simulink model "numerical_model"  (R2021a)
settings: Solver=VariableStepAuto  StartTime=0.0  StopTime=100  RelTol=1e-6
values from neighbouring files (symbols this model uses):
  d_f = 0.1*[1 1 1].'    [working_numerlical_sim_sys_param.m]
  d_tau = 0.1*[1 1 1].'    [working_numerlical_sim_sys_param.m]
  g = 9.81    [working_numerlical_sim_sys_param.m]
  Gamma = 0.1*eye(6)    [working_numerlical_sim_sys_param.m]
  J = [0.0169572, 0 0; 0 0.0169572 0; 0 0 0.0338078]    [working_numerlical_sim_sys_param.m]
  Jv0 = 0.8*[J(1,1) J(2,2) J(3,3) J(1,2) J(2,3) J(1,3)].'    [working_numerlical_sim_sys_param.m]
  k1 = 0.4    [working_numerlical_sim_sys_param.m]
  k2 = 0.5    [working_numerlical_sim_sys_param.m]
  k3 = 0.5    [working_numerlical_sim_sys_param.m]
  k4 = 2    [working_numerlical_sim_sys_param.m]
  k5 = 1    [working_numerlical_sim_sys_param.m]
  k_dtau = 1    [working_numerlical_sim_sys_param.m]
  k_psi1 = 1    [working_numerlical_sim_sys_param.m]
  k_psi2 = 1    [working_numerlical_sim_sys_param.m]
  lambda = 86    [working_numerlical_sim_sys_param.m]
  m = quadrotor_mass+link0_mass+link1_mass    (= 1.8)    [working_numerlical_sim_sys_param.m]
  m0 = 0.9*m    (= 1.62)    [working_numerlical_sim_sys_param.m]
  omega_0 = 0*[0.1 -0.1 0.1].'    [working_numerlical_sim_sys_param.m]
  p_0 = [-0.1 0.1 -0.9].'    [working_numerlical_sim_sys_param.m]
  R_0 = eye(3)    [working_numerlical_sim_sys_param.m]
  v_0 = [0 0 0].'    [working_numerlical_sim_sys_param.m]
settings Model: Creator=Awais  LastModifiedBy=awais
settings SolverCC: AlgebraicLoopSolver=TrustRegion
settings DebuggingCC: SFMachineParentedDataDiag=warning
settings ExplorerConfigSet: InternalSimMechanicsExplorerSettings="<ExplorerConfiguration><canonicalview>aerospace</canonicalview><AnimationSetting><BasePlaybackSpeed>1.0</BasePlaybackSpeed><PlaybackSpeedFactor>1.0</PlaybackSpeedFactor></AnimationSetting><TilePanel><TileInfo><Tiles Columns=\"1\" Count=\"1\" Rows=\"1\"><Column Weight=\"1\"/><Row Weight=\"1\"/><Tile Height=\"1\" Width=\"1\" X=\"0\" Y=\"0\"/></Tiles></TileInfo><SceneInfo><SceneViewer><BGColor><R>1</R><G>1</G><B>1</B></BGColor><Camera><DoPerspective>off</DoPerspective><Position><X>9.64020367718573112</X><Y>-9.14802033169267048</Y><Z>-6.8961967369270063</Z></Position><Center><X>1.75390707402820034</X><Y>-2.22859187648804102</Y><Z>3.98852762898917668</Z></Center><Up><X>-0.508228210550880632</X><Y>0.511125189703023119</Y><Z>-0.69314870442878207</Z></Up><ViewLimDist>1</ViewLimDist><YLim>6.89917364541416234</YLim><XLim>10.5845954884453661</XLim></Camera></SceneViewer></SceneInfo></TilePanel><MechEditorPanel><Cameras/><GfxPanelCameraMap/><VideoCreator><PlaybackSpeedRatio>1.0</PlaybackSpeedRatio><FrameRate>30</FrameRate><VideoFormat>Motion JPEG AVI</VideoFormat><FrameSize>auto</FrameSize></VideoCreator></MechEditorPanel></ExplorerConfiguration>"

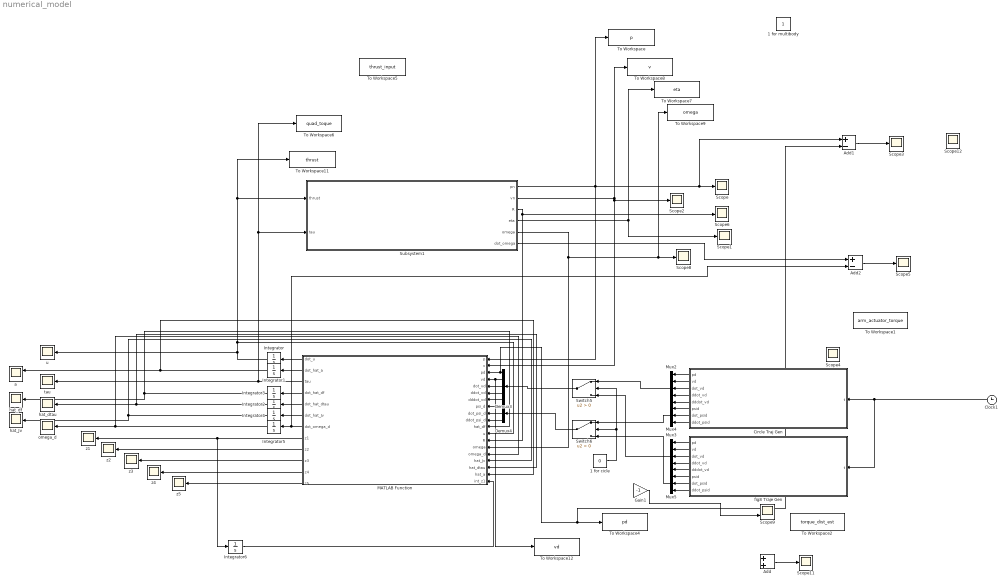
== system numerical_model ==
  1 for cicle : Constant  Value=0
  1 for multibody : Constant
  Add : Sum
  Add1 : Sum  Inputs=+-
  Add2 : Sum  Inputs=+-
  Circle Traj Gen : MATLAB Function  TreatAsAtomicUnit=on
  Clock1 : Clock
  Demux3 : Demux  Outputs=5
  Demux4 : Demux  Outputs=3
  Gain1 : Gain  Gain=-1
  Integrator : Integrator  InitialCondition=m*g
  Integrator1 : Integrator  InitialCondition=1/m0
  Integrator2 : Integrator
  Integrator3 : Integrator
  Integrator4 : Integrator  InitialCondition=Jv0
  Integrator5 : Integrator  InitialCondition=[0 0 0]
  Integrator6 : Integrator
  MATLAB Function : MATLAB Function  TreatAsAtomicUnit=on
  Mux2 : Mux  Inputs=5
  Mux3 : Mux  Inputs=5
  Mux4 : Mux  Inputs=3
  Mux5 : Mux  Inputs=3
  Scope{,1..6,8,11} (9 alike) : Scope
  Scope12 : Scope  NumInputPorts=2
  Scope9 : Scope  NumInputPorts=2
  Subsystem1 : Subsystem
  Switch5 : Switch  Criteria=u2 > Threshold
  Switch6 : Switch  Criteria=u2 > Threshold
  To Workspace : ToWorkspace  VariableName=p  SaveFormat=Structure With Time  SampleTime=-1
  To Workspace1 : ToWorkspace  VariableName=arm_actuator_torque  SaveFormat=Structure With Time  SampleTime=-1
  To Workspace11 : ToWorkspace  VariableName=thrust  SaveFormat=Structure With Time  SampleTime=-1
  To Workspace12 : ToWorkspace  VariableName=vd  SaveFormat=Structure With Time  SampleTime=-1
  To Workspace2 : ToWorkspace  VariableName=torque_dist_est  SaveFormat=Structure With Time  SampleTime=-1
  To Workspace4 : ToWorkspace  VariableName=pd  SaveFormat=Structure With Time  SampleTime=-1
  To Workspace5 : ToWorkspace  VariableName=thrust_input  SaveFormat=Structure With Time  SampleTime=-1
  To Workspace6 : ToWorkspace  VariableName=quad_toque  SaveFormat=Structure With Time  SampleTime=-1
  To Workspace7 : ToWorkspace  VariableName=eta  SaveFormat=Structure With Time  SampleTime=-1
  To Workspace8 : ToWorkspace  VariableName=v  SaveFormat=Structure With Time  SampleTime=-1
  To Workspace9 : ToWorkspace  VariableName=omega  SaveFormat=Structure With Time  SampleTime=-1
  a : Scope  NumInputPorts=2
  fig8 Traje Gen : MATLAB Function  TreatAsAtomicUnit=on
  hat_Jv : Scope
  hat_df : Scope
  hat_dtau : Scope
  omega_d : Scope
  tau : Scope
  u : Scope
  z{1..5} (5 alike) : Scope
  wires:
  MATLAB Function/1(dot_u) -> Integrator/1
  Integrator/1 -> u/1, To Workspace11/1, Subsystem1/1(thrust), MATLAB Function/12(u)
  MATLAB Function/2(dot_hat_a) -> Integrator1/1
  MATLAB Function/5(dot_hat_dtau) -> Integrator2/1
  MATLAB Function/3(tau) -> To Workspace6/1, Subsystem1/2(tau), tau/1
  Clock1/1 -> fig8 Traje Gen/1(t), Circle Traj Gen/1(t)
  Gain1/1 -> Scope9/2
  Circle Traj Gen/1(pd) -> Mux2/1
  Circle Traj Gen/2(vd) -> Mux2/2
  Circle Traj Gen/3(dot_vd) -> Mux2/3
  Circle Traj Gen/4(ddot_vd) -> Mux2/4
  Circle Traj Gen/5(dddot_vd) -> Mux2/5
  Mux2/1 -> Switch5/1
  Demux3/5 -> MATLAB Function/7(dddot_vd)
  Demux3/4 -> MATLAB Function/6(ddot_vd)
  Demux3/3 -> MATLAB Function/5(dot_vd)
  Demux3/1 -> Add1/2, To Workspace4/1, MATLAB Function/3(pd)
  Switch5/1 -> Demux3/1
  1 for cicle/1 -> Switch6/2, Switch5/2
  fig8 Traje Gen/1(pd) -> Mux3/1
  fig8 Traje Gen/2(vd) -> Mux3/2
  fig8 Traje Gen/3(dot_vd) -> Mux3/3
  fig8 Traje Gen/4(ddot_vd) -> Mux3/4
  fig8 Traje Gen/5(dddot_vd) -> Mux3/5
  Mux3/1 -> Switch5/3
  Circle Traj Gen/6(psid) -> Mux4/1
  Circle Traj Gen/7(dot_psid) -> Mux4/2
  Circle Traj Gen/8(ddot_psid) -> Mux4/3
  Mux4/1 -> Switch6/1
  fig8 Traje Gen/6(psid) -> Mux5/1
  fig8 Traje Gen/7(dot_psid) -> Mux5/2
  fig8 Traje Gen/8(ddot_psid) -> Mux5/3
  Mux5/1 -> Switch6/3
  Demux4/1 -> MATLAB Function/8(psi_d)
  Demux4/2 -> MATLAB Function/9(dot_psi_d)
  Demux4/3 -> MATLAB Function/10(ddot_psi_d)
  Switch6/1 -> Demux4/1
  Add/1 -> Scope11/1
  Demux3/2 -> To Workspace12/1, MATLAB Function/4(vd)
  MATLAB Function/4(dot_hat_df) -> Integrator3/1
  Integrator3/1 -> hat_df/1, MATLAB Function/11(hat_df)
  Integrator1/1 -> a/1, MATLAB Function/18(hat_a)
  MATLAB Function/8(z1) -> z1/1, Integrator6/1
  MATLAB Function/9(z2) -> z2/1
  MATLAB Function/10(z3) -> z3/1
  MATLAB Function/11(z4) -> z4/1
  Integrator2/1 -> hat_dtau/1, MATLAB Function/17(hat_dtau)
  MATLAB Function/6(dot_hat_Jv) -> Integrator4/1
  MATLAB Function/7(dot_omega_d) -> Add2/2, Integrator5/1
  MATLAB Function/12(z5) -> z5/1
  Integrator5/1 -> omega_d/1, MATLAB Function/15(omega_d)
  Subsystem1/1(pn) -> To Workspace/1, Add1/1, Scope/1, MATLAB Function/1(p)
  Subsystem1/2(vn) -> MATLAB Function/2(v), Scope2/1, To Workspace8/1
  Subsystem1/3(R) -> Scope6/1, MATLAB Function/13(R)
  Subsystem1/5(omega) -> To Workspace9/1, Scope8/1, MATLAB Function/14(omega)
  Subsystem1/4(eta) -> Scope1/1, To Workspace7/1
  Add1/1 -> Scope3/1
  Integrator6/1 -> MATLAB Function/19(int_z1)
  Add2/1 -> Scope5/1
  Subsystem1/6(dot_omega) -> Add2/1
  Integrator4/1 -> MATLAB Function/16(hat_Jv), hat_Jv/1

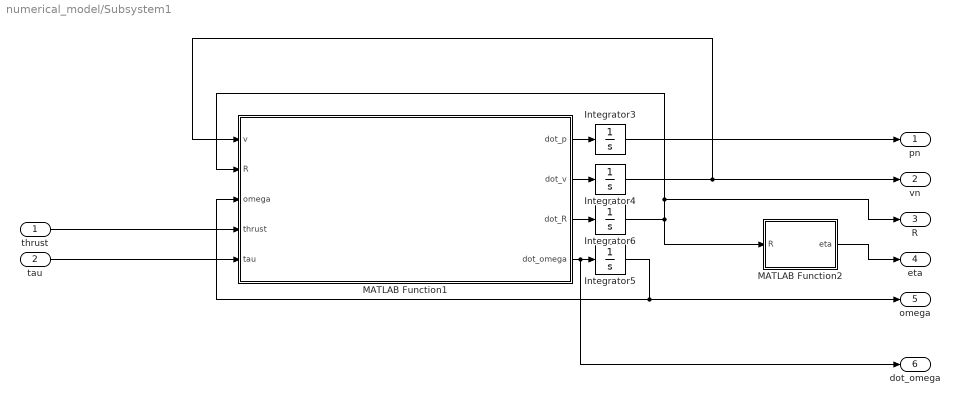
== system numerical_model/Subsystem1 ==
  thrust : Inport
  tau : Inport  Port=2
  Integrator3 : Integrator  InitialCondition=p_0
  Integrator4 : Integrator  InitialCondition=v_0
  Integrator5 : Integrator  InitialCondition=omega_0
  Integrator6 : Integrator  InitialCondition=R_0
  MATLAB Function1 : MATLAB Function  TreatAsAtomicUnit=on
  MATLAB Function2 : MATLAB Function  TreatAsAtomicUnit=on
  pn : Outport
  vn : Outport  Port=2
  R : Outport  Port=3
  eta : Outport  Port=4
  omega : Outport  Port=5
  dot_omega : Outport  Port=6
  wires:
  MATLAB Function1/4(dot_omega) -> dot_omega/1, Integrator5/1
  MATLAB Function1/3(dot_R) -> Integrator6/1
  Integrator6/1 -> MATLAB Function1/2(R), R/1, MATLAB Function2/1(R)
  MATLAB Function1/1(dot_p) -> Integrator3/1
  MATLAB Function1/2(dot_v) -> Integrator4/1
  Integrator4/1 -> vn/1, MATLAB Function1/1(v)
  Integrator3/1 -> pn/1
  Integrator5/1 -> omega/1, MATLAB Function1/3(omega)
  tau/1 -> MATLAB Function1/5(tau)
  thrust/1 -> MATLAB Function1/4(thrust)
  MATLAB Function2/1(eta) -> eta/1

== matlab function numerical_model/Subsystem1/MATLAB Function1 ==
  data: v input; dot_p output; R input; omega input; thrust input; tau input; dot_v output; dot_R output; dot_omega output; m parameter; g parameter; J parameter; d_f parameter; d_tau parameter
function [dot_p, dot_v, dot_R, dot_omega] = fcn(v,R,omega,thrust,tau,m, g, J, d_f, d_tau)
n3=[0 0 1].';
dot_p = v;
dot_v = g*n3 - R*n3*thrust/m + d_f;
dot_R = R*skew(omega);
dot_omega = J^-1 * (- skew(omega)*J*omega + tau + d_tau);

== matlab function numerical_model/Subsystem1/MATLAB Function2 ==
  data: R input; eta output
function eta = q2eul(R)
eta=flip(rotm2eul(R));

== matlab function numerical_model/Circle Traj Gen ==
  data: t input; pd output; vd output; dot_vd output; ddot_vd output; dddot_vd output; psid output; dot_psid output; ddot_psid output
function [pd, vd, dot_vd, ddot_vd, dddot_vd, psid, dot_psid, ddot_psid] = fcn(t)

T = 6;%Time to complete one circle loop 
w = 2*pi/T;
pd = [-0.8 0.9 -1].';
vd = [0 0 0].';
dot_vd = vd;
ddot_vd = vd;
dddot_vd = vd;


pd(2) = sin(w*t);
vd(2) = cos(w*t)*w;
dot_vd(2) = -sin(w*t)*w^2;
ddot_vd(2) = -cos(w*t)*w^3;
dddot_vd(2) = sin(w*t)*w^4;

pd(1) = cos(w*t);
vd(1) = -sin(w*t)*w;
dot_vd(1) = -cos(w*t)*w^2;
ddot_vd(1) = sin(w*t)*w^3;
dddot_vd(1) = cos(w*t)*w^4;

% pd(1) = 0;
% vd(1) = 0;
% dot_vd(1) = 0;
% ddot_vd(1) = 0;
% dddot_vd(1) = 0;
% 
% pd(2) = 0;
% vd(2) = 0;
% dot_vd(2) = 0;
% ddot_vd(2) = 0;
% dddot_vd(2) = 0;

pd(3) = -1;
vd(3) = 0;
dot_vd(3) = 0;
ddot_vd(3) = 0;
dddot_vd(3) = 0;

psid = 0;
dot_psid = 0;
ddot_psid = 0;

== matlab function numerical_model/fig8 Traje Gen ==
  data: t input; pd output; vd output; dot_vd output; ddot_vd output; dddot_vd output; psid output; dot_psid output; ddot_psid output
function [pd, vd, dot_vd, ddot_vd, dddot_vd, psid, dot_psid, ddot_psid] = fcn(t)

T = 6;%Time to complete one circle loop 
w = 2*pi/T;

A = 1.5;
B = A/2;
pd = [0 0 0].';
vd = pd;
dot_vd = pd;
ddot_vd = pd;
dddot_vd = pd;


pd(1) = A*sin(w*t);
vd(1) = A*cos(w*t)*w;
dot_vd(1) = -A*sin(w*t)*w^2;
ddot_vd(1) = -A*cos(w*t)*w^3;
dddot_vd(1) = -A*sin(w*t)*w^4;

pd(2) = B*sin(2*w*t);
vd(2) = B*cos(2*w*t)*2*w;
dot_vd(2) = -B*sin(2*w*t)*(2*w)^2;
ddot_vd(2) = -B*cos(2*w*t)*(2*w)^3;
dddot_vd(2) = B*sin(2*w*t)*(2*w)^4;

pd(3) = -1;
vd(3) = 0;
dot_vd(3) = 0;
ddot_vd(3) = 0;
dddot_vd(3) = 0;

psid = 0;
dot_psid = 0;
ddot_psid = 0;

== matlab function numerical_model/MATLAB Function ==
  data: p input; v input; pd input; dot_u output; dot_hat_a output; vd input; dot_vd input; ddot_vd input; dddot_vd input; psi_d input; dot_psi_d input; ddot_psi_d input; hat_df input; u input; R input; omega input; omega_d input; hat_Jv input; hat_dtau input; tau output; dot_hat_df output; dot_hat_dtau output; dot_hat_Jv output; k_dtau parameter; k1 parameter; k2 parameter; k3 parameter; k4 parameter; g parameter; J parameter; k_psi1 parameter; k_psi2 parameter; dot_omega_d output; hat_a input; lambda parameter; z1 output; z2 output; z3 output; z4 output; z5 output; Gamma parameter; k5 parameter; int_z1 input; d_tau parameter; m parameter; d_f parameter
function [dot_u, dot_hat_a, tau, dot_hat_df, dot_hat_dtau, dot_hat_Jv, dot_omega_d, z1, z2, z3, z4, z5] = fcn(p, v, pd, vd,  dot_vd, ddot_vd, dddot_vd, psi_d, dot_psi_d, ddot_psi_d, hat_df, u, R, omega, omega_d, hat_Jv, hat_dtau, k_dtau, k1, k2, k3, k4, g, J, k_psi1, k_psi2, hat_a, lambda, Gamma, k5, int_z1, d_tau, m, d_f)
n1 = [1 0 0].';
n2 = [0 1 0].';
n3 = [0 0 1].';
Sw = skew(omega);

I=eye(3);

if hat_a < 0.01
    hat_a = 0.01;
end
if u < 0.1
    u = 0.1;
end
hat_df = d_f;
hat_a = 1/m;
k = k1^2 + k2^2 + 3*k1*k2 + k2*k3 + k3*k1 + 3*eye(1);

z1 = p-pd;
z2 = v - vd + k1*z1;
z3 = g*n3 - hat_a*u*R*n3 + hat_df - dot_vd + (1*eye(1)-k1^2)*z1 + (k1+k2)*z2;

sigma1 = (k1*(k1^2-1)-k2-k1)*z1 + (2*eye(1)-k2*(k1+k2)-k1^2)*z2 + (k1+k2+k3)*z3 - ddot_vd;
sigma2 = z2 + (k1+k2)*z3;

z4 = -hat_a*u*Sw*n3 + (I-n3*n3.')*R.'*(sigma1 + sigma2);

%dot_hat_a = -(1/lambda)*u*sigma2.'*n3;
dot_hat_a = 0;

%dot_hat_df = sigma2 + k*R*(I-n3*n3.')*R.'*z4;
dot_hat_df = 0;

dot_u = (1/hat_a)*( -dot_hat_a*u + n3.'*R.'*(sigma1 + sigma2));

bar_sigma1 = (k1^2 + k1*k2 + k2^2 - 2*eye(1))*(z1 - z3 + k2*z2) - (- k1^3 + 2*k1 + k2)*(z2 - k1*z1)- dddot_vd...
    +(k1 + k2 + k3)*(-(hat_a*dot_u +dot_hat_a*u)*R*n3 - hat_a*u*R*Sw*n3 + dot_hat_df + sigma1 - z2 -k3*z3) ;
bar_sigma2 = z3 - z1 - k2*z2 + (k1 + k2)*(-z2 - k3*z3) + (k1 + k2)*(-(hat_a*dot_u +dot_hat_a*u)*R*n3 - hat_a*u*R*Sw*n3 + dot_hat_df + sigma1);

auSwn3 = R.'*z3 + k4*z4 + k*(I-n3*n3.')*R.'*z3 - (hat_a*dot_u +dot_hat_a*u)*Sw*n3 ...
    + (I-n3*n3.')*Sw.'*R.'*(sigma1 + sigma2) + (I-n3*n3.')*R.'*(bar_sigma1 + bar_sigma2);

dot_omega_d = [0 0 0].';

dot_omega_d(1) = -  n2.'*(1/(hat_a*u) )*auSwn3;
dot_omega_d(2) =  n1.'*(1/(hat_a*u) )*auSwn3;

eta = flip(rotm2eul(R));
phi = eta(1);
theta = eta(2);
psi = eta(3);
dot_eta = [1, (sin(phi)*sin(theta))/cos(theta), (cos(phi)*sin(theta))/cos(theta);... 
           0,                         cos(phi),                        -sin(phi);...
           0,              sin(phi)/cos(theta),              cos(phi)/cos(theta)]*omega;
dot_phi = dot_eta(1);
dot_theta = dot_eta(2);
dot_psi = dot_eta(3);
       
epsilon_1 = psi - psi_d;
alpha_psi1 = dot_psi_d - k_psi1 * epsilon_1;
epsilon_2 = dot_psi - alpha_psi1;
dot_alpha_psi1 = ddot_psi_d - k_psi1*(dot_psi- dot_psi_d);
n3dot_W_eta = [0 (cos(phi)*cos(theta)*dot_phi + sin(phi)*sin(theta)*dot_theta)/(cos(theta)^2) (-sin(phi)*cos(theta)*dot_phi + cos(phi)*sin(theta)*dot_theta)/(cos(theta)^2)];

dot_omega_d(3) = (cos(theta)/cos(phi))*(dot_alpha_psi1 - epsilon_1 - k_psi2*epsilon_2 - n3dot_W_eta*omega - sin(phi)*dot_omega_d(2)/cos(theta));
%dot_omega_d(3) = 0;

% Phi_omega = [0  -omega(2)*omega(3)  omega(2)*omega(3) -omega(1)*omega(3) (omega(2)^2 - omega(3)^2) omega(1)*omega(2);...
%     omega(1)*omega(3)  0  -omega(1)*omega(3) omega(2)*omega(3) -omega(1)*omega(2) (omega(3)^2 - omega(1)^2);...
%     -omega(1)*omega(2) omega(1)*omega(2) 0 (omega(1)^2-omega(2)^2) omega(1)*omega(3) -omega(2)*omega(3)];
%     
% 
% Psi_dot_omega_d = [dot_omega_d(1) 0 0 dot_omega_d(2) 0 dot_omega_d(3);...
%                    0 dot_omega_d(2) 0 dot_omega_d(1) dot_omega_d(3) 0;...
%                    0 0 dot_omega_d(3) 0 dot_omega_d(2) dot_omega_d(1)];
%                
% z5 = omega - omega_d;

%tau = (Phi_omega + Psi_dot_omega_d)*hat_Jv - k5*z5 - hat_dtau;
tau = J*dot_omega_d+Sw*J*omega-d_tau;
dot_hat_Jv = 0;
dot_hat_dtau = 0;
% dot_hat_Jv = -Gamma*(Phi_omega + Psi_dot_omega_d).'*z5;
% 
% dot_hat_dtau = k_dtau*z5;
z5 = omega - omega_d;




% hat_dtau = z_dtau + k_dtau*J*omega;
% 
% 
% tau = J*dot_omega_d + cross(omega, J*omega) - hat_dtau;
% 
% 
% dot_z_dtau = -k_dtau * hat_dtau - k_dtau * (-cross(omega,J*omega)+tau);
tau = [tau(1) tau(2) tau(3)].';
